simulink model "target_driver_2022_Ctrl_v_2_4_landing_2017a"  (R2024b)
settings: Solver=FixedStepDiscrete  StartTime=0.0  StopTime=13  FixedStep=0.0001  RelTol=1e-3  EnableMultiTasking=on
values from neighbouring files (symbols this model uses):
  A = gamma_2*gamma_3*Thrust_desired    [force2voltage.m]
  a2_lb = -0.25    [target_driver_setup_2022_Ctrl_V_2_4.m]    (also in target_driver_setup_2022_Ctrl_V_2_4_geometric.m; target_driver_setup_mpc_12msdelay.m; target_driver_setup_mpc_andWLQP.m)
  a2_openloop = -0    (= 0)    [target_driver_setup_2022_Ctrl_V_2_4.m]    (also in target_driver_setup_2022_Ctrl_V_2_4_geometric.m; target_driver_setup_mpc_12msdelay.m; target_driver_setup_mpc_andWLQP.m)
  a2_ub = 0.25    [target_driver_setup_2022_Ctrl_V_2_4.m]    (also in target_driver_setup_2022_Ctrl_V_2_4_geometric.m; target_driver_setup_mpc_12msdelay.m; target_driver_setup_mpc_andWLQP.m)
  adaptive_flag = 0    [target_driver_setup_2022_Ctrl_V_2_4.m]    (also in target_driver_setup_2022_Ctrl_V_2_4_geometric.m; target_driver_setup_mpc_12msdelay.m = 1; target_driver_setup_mpc_andWLQP.m = 1)
  adaptive_gain = [gamma_adaptive, adaptive_roll_limit, adaptive_pitch_limit, adaptive_yaw_limit, c_2_adaptive, gamma_lateral_adaptive, adaptive_x_limit, adaptive_y_limit, adaptive_z_limit, c_1_adaptive]    [target_driver_setup_2022_Ctrl_V_2_4.m]    (also in target_driver_setup_2022_Ctrl_V_2_4_geometric.m; target_driver_setup_mpc_12msdelay.m; target_driver_setup_mpc_andWLQP.m)
  adaptive_lateral_flag = 0    [target_driver_setup_2022_Ctrl_V_2_4.m]    (also in target_driver_setup_2022_Ctrl_V_2_4_geometric.m; target_driver_setup_mpc_12msdelay.m = 1; target_driver_setup_mpc_andWLQP.m = 1)
  adaptive_pitch_init = 0    [target_driver_setup_2022_Ctrl_V_2_4.m]    (also in target_driver_setup_2022_Ctrl_V_2_4_geometric.m; target_driver_setup_mpc_12msdelay.m; target_driver_setup_mpc_andWLQP.m)
  adaptive_pitch_limit = 0.1/(scale^2)    (= 1e-07)    [target_driver_setup_2022_Ctrl_V_2_4.m]    (also in target_driver_setup_2022_Ctrl_V_2_4_geometric.m = 3e-07; target_driver_setup_mpc_12msdelay.m; target_driver_setup_mpc_andWLQP.m)
  adaptive_pitch_limit_low = -adaptive_pitch_limit    (= -1e-07)    [target_driver_setup_2022_Ctrl_V_2_4.m]    (also in target_driver_setup_2022_Ctrl_V_2_4_geometric.m = -3e-07; target_driver_setup_mpc_12msdelay.m; target_driver_setup_mpc_andWLQP.m)
  adaptive_roll_init = 0    [target_driver_setup_2022_Ctrl_V_2_4.m]    (also in target_driver_setup_2022_Ctrl_V_2_4_geometric.m; target_driver_setup_mpc_12msdelay.m; target_driver_setup_mpc_andWLQP.m)
  adaptive_roll_limit = 0.3/(scale^2)    (= 3e-07)    [target_driver_setup_2022_Ctrl_V_2_4.m]    (also in target_driver_setup_2022_Ctrl_V_2_4_geometric.m; target_driver_setup_mpc_12msdelay.m; target_driver_setup_mpc_andWLQP.m)
  adaptive_roll_limit_low = -adaptive_roll_limit    (= -3e-07)    [target_driver_setup_2022_Ctrl_V_2_4.m]    (also in target_driver_setup_2022_Ctrl_V_2_4_geometric.m; target_driver_setup_mpc_12msdelay.m; target_driver_setup_mpc_andWLQP.m)
  adaptive_x_init = 0    [target_driver_setup_2022_Ctrl_V_2_4.m]    (also in target_driver_setup_2022_Ctrl_V_2_4_geometric.m; target_driver_setup_mpc_12msdelay.m; target_driver_setup_mpc_andWLQP.m)
  adaptive_x_limit = 0.15/(scale)    (= 0.00015)    [target_driver_setup_2022_Ctrl_V_2_4.m]    (also in target_driver_setup_2022_Ctrl_V_2_4_geometric.m = 7.5e-05; target_driver_setup_mpc_12msdelay.m; target_driver_setup_mpc_andWLQP.m)
  adaptive_x_limit_low = -adaptive_x_limit    (= -0.00015)    [target_driver_setup_2022_Ctrl_V_2_4.m]    (also in target_driver_setup_2022_Ctrl_V_2_4_geometric.m = -7.5e-05; target_driver_setup_mpc_12msdelay.m; target_driver_setup_mpc_andWLQP.m)
  adaptive_y_init = 0    [target_driver_setup_2022_Ctrl_V_2_4.m]    (also in target_driver_setup_2022_Ctrl_V_2_4_geometric.m; target_driver_setup_mpc_12msdelay.m; target_driver_setup_mpc_andWLQP.m)
  adaptive_y_limit = 0.15/(scale)    (= 0.00015)    [target_driver_setup_2022_Ctrl_V_2_4.m]    (also in target_driver_setup_2022_Ctrl_V_2_4_geometric.m = 7.5e-05; target_driver_setup_mpc_12msdelay.m; target_driver_setup_mpc_andWLQP.m)
  adaptive_y_limit_low = -adaptive_y_limit    (= -0.00015)    [target_driver_setup_2022_Ctrl_V_2_4.m]    (also in target_driver_setup_2022_Ctrl_V_2_4_geometric.m = -7.5e-05; target_driver_setup_mpc_12msdelay.m; target_driver_setup_mpc_andWLQP.m)
  adaptive_yaw_init = 0    [target_driver_setup_2022_Ctrl_V_2_4.m]    (also in target_driver_setup_2022_Ctrl_V_2_4_geometric.m; target_driver_setup_mpc_12msdelay.m; target_driver_setup_mpc_andWLQP.m)
  adaptive_yaw_limit = 0.035/(scale^2)    (= 3.5e-08)    [target_driver_setup_2022_Ctrl_V_2_4.m]    (also in target_driver_setup_2022_Ctrl_V_2_4_geometric.m; target_driver_setup_mpc_12msdelay.m; target_driver_setup_mpc_andWLQP.m)
  adaptive_yaw_limit_low = -adaptive_yaw_limit    (= -3.5e-08)    [target_driver_setup_2022_Ctrl_V_2_4.m]    (also in target_driver_setup_2022_Ctrl_V_2_4_geometric.m; target_driver_setup_mpc_12msdelay.m; target_driver_setup_mpc_andWLQP.m)
  adaptive_z_init = 0/scale    (= 0)    [target_driver_setup_2022_Ctrl_V_2_4.m]    (also in target_driver_setup_2022_Ctrl_V_2_4_geometric.m; target_driver_setup_mpc_12msdelay.m; target_driver_setup_mpc_andWLQP.m)
  adaptive_z_limit = 0.20/(scale)    (= 0.0002)    [target_driver_setup_2022_Ctrl_V_2_4.m]    (also in target_driver_setup_2022_Ctrl_V_2_4_geometric.m = 0.0008; target_driver_setup_mpc_12msdelay.m = 0.0008; target_driver_setup_mpc_andWLQP.m = 0.0008)
  adaptive_z_limit_low = -adaptive_z_limit/1    (= -0.0002)    [target_driver_setup_2022_Ctrl_V_2_4.m]    (also in target_driver_setup_2022_Ctrl_V_2_4_geometric.m = -0.0008; target_driver_setup_mpc_12msdelay.m = -0.0008; target_driver_setup_mpc_andWLQP.m = -0.0008)
  att_s = 500    [target_driver_setup_2022_Ctrl_V_2_4.m]    (also in target_driver_setup_2022_Ctrl_V_2_4_geometric.m; target_driver_setup_mpc_12msdelay.m; target_driver_setup_mpc_andWLQP.m)
  b_1_d_desired = [1,0,0]    [target_driver_setup_2022_Ctrl_V_2_4.m]    (also in target_driver_setup_2022_Ctrl_V_2_4_geometric.m; target_driver_setup_mpc_12msdelay.m; target_driver_setup_mpc_andWLQP.m)
  closedloop_flag = 1    [target_driver_setup_2022_Ctrl_V_2_4.m]    (also in target_driver_setup_2022_Ctrl_V_2_4_geometric.m = 0; target_driver_setup_mpc_12msdelay.m = 0; target_driver_setup_mpc_andWLQP.m = 0)
  control_gain = [k_x,k_v, k_R, k_Omega, k_z, k_vz, k_Rx]    [target_driver_setup_2022_Ctrl_V_2_4.m]    (also in target_driver_setup_2022_Ctrl_V_2_4_geometric.m = [k_x,k_v,k_R,k_Omega_pitch,k_Omega_roll,k_z,k_vz,k_Rx]; target_driver_setup_mpc_12msdelay.m = [k_x, k_v, k_R, k_Omega, k_z, k_vz, k_Rx,                  k; target_driver_setup_mpc_andWLQP.m = [k_x, k_v, k_R, k_Omega, k_z, k_vz, k_Rx,                  k)
  delay = delay-vicon_sample_cycle/2    [target_driver_setup_2022_Ctrl_V_2_4.m]    (also in target_driver_setup_2022_Ctrl_V_2_4_geometric.m; target_driver_setup_mpc_12msdelay.m; target_driver_setup_mpc_andWLQP.m)
  drv_amp = abs((vleft_p2p-vright_p2p))/2+min(vleft_p2p,vright_p2p)    [Wing_traj_to_Voltage.m]    (also in force2voltage.m; target_driver_setup_2022_Ctrl_V_2_4.m = 160; target_driver_setup_2022_Ctrl_V_2_4_geometric.m = 110; target_driver_setup_mpc_12msdelay.m = 150)
  drv_bias = max_drv_bias    (= 300)    [target_driver_setup_2022_Ctrl_V_2_4.m]    (also in target_driver_setup_2022_Ctrl_V_2_4_geometric.m = 200; target_driver_setup_mpc_12msdelay.m = 200; target_driver_setup_mpc_andWLQP.m = 200)
  drv_pitch_left = vleft_pitch    [Wing_traj_to_Voltage.m]    (also in force2voltage.m = 0; target_driver_setup_2022_Ctrl_V_2_4.m = 0; target_driver_setup_2022_Ctrl_V_2_4_geometric.m = 9.05; target_driver_setup_mpc_12msdelay.m = 9.05)
  drv_pitch_right = vright_pitch    [Wing_traj_to_Voltage.m]    (also in force2voltage.m = 0; target_driver_setup_2022_Ctrl_V_2_4.m = 0; target_driver_setup_2022_Ctrl_V_2_4_geometric.m = 9.05; target_driver_setup_mpc_12msdelay.m = 9.05)
  drv_roll = (vleft_p2p-vright_p2p)/4    [Wing_traj_to_Voltage.m]    (also in force2voltage.m; target_driver_setup_2022_Ctrl_V_2_4.m = -2; target_driver_setup_2022_Ctrl_V_2_4_geometric.m = -0.001; target_driver_setup_mpc_12msdelay.m = -0.001)
  f_fin = f    (= 155)    [target_driver_setup_2022_Ctrl_V_2_4.m]    (also in target_driver_setup_2022_Ctrl_V_2_4_geometric.m; target_driver_setup_mpc_12msdelay.m; target_driver_setup_mpc_andWLQP.m)
  f_int = f    (= 155)    [target_driver_setup_2022_Ctrl_V_2_4.m]    (also in target_driver_setup_2022_Ctrl_V_2_4_geometric.m; target_driver_setup_mpc_12msdelay.m; target_driver_setup_mpc_andWLQP.m)
  g = 9.8    [target_driver_setup_2022_Ctrl_V_2_4.m]    (also in target_driver_setup_2022_Ctrl_V_2_4_geometric.m; target_driver_setup_mpc_12msdelay.m; target_driver_setup_mpc_andWLQP.m = 9.81; test_full_attitude_mpc.m = 9.81)
  I_moment_vec = [Ixx, Iyy, Izz]    [target_driver_setup_2022_Ctrl_V_2_4.m]    (also in target_driver_setup_2022_Ctrl_V_2_4_geometric.m; target_driver_setup_mpc_12msdelay.m; target_driver_setup_mpc_andWLQP.m)
  landing_flag = 0    [target_driver_setup_2022_Ctrl_V_2_4.m]    (also in target_driver_setup_2022_Ctrl_V_2_4_geometric.m; target_driver_setup_mpc_12msdelay.m; target_driver_setup_mpc_andWLQP.m)
  landing_parameter = [start_delay+T,transition_rate, rising_time, falling_time, landing_rising_time, landing_z_decrease, landing_y_decrease, landing_x_decrease]    [target_driver_setup_2022_Ctrl_V_2_4.m]    (also in target_driver_setup_2022_Ctrl_V_2_4_geometric.m; target_driver_setup_mpc_12msdelay.m; target_driver_setup_mpc_andWLQP.m)
  low_bound = -8    [target_driver_setup_2022_Ctrl_V_2_4.m]    (also in target_driver_setup_2022_Ctrl_V_2_4_geometric.m = -5; target_driver_setup_mpc_12msdelay.m = -10; target_driver_setup_mpc_andWLQP.m = -10)
  low_bound_eR = -0.8    [target_driver_setup_2022_Ctrl_V_2_4.m]    (also in target_driver_setup_2022_Ctrl_V_2_4_geometric.m = -1.2; target_driver_setup_mpc_12msdelay.m = -1.2; target_driver_setup_mpc_andWLQP.m = -1.2)
  low_bound_vx = -0.5    [target_driver_setup_2022_Ctrl_V_2_4.m]    (also in target_driver_setup_2022_Ctrl_V_2_4_geometric.m; target_driver_setup_mpc_12msdelay.m; target_driver_setup_mpc_andWLQP.m)
  low_bound_vy = -0.5    [target_driver_setup_2022_Ctrl_V_2_4.m]    (also in target_driver_setup_2022_Ctrl_V_2_4_geometric.m; target_driver_setup_mpc_12msdelay.m; target_driver_setup_mpc_andWLQP.m)
  low_bound_vz = -0.5    [target_driver_setup_2022_Ctrl_V_2_4.m]    (also in target_driver_setup_2022_Ctrl_V_2_4_geometric.m; target_driver_setup_mpc_12msdelay.m; target_driver_setup_mpc_andWLQP.m)
  low_bound_x = -0.06    [target_driver_setup_2022_Ctrl_V_2_4.m]    (also in target_driver_setup_2022_Ctrl_V_2_4_geometric.m = -0.1; target_driver_setup_mpc_12msdelay.m = -0.6; target_driver_setup_mpc_andWLQP.m = -0.6)
  low_bound_y = -0.06    [target_driver_setup_2022_Ctrl_V_2_4.m]    (also in target_driver_setup_2022_Ctrl_V_2_4_geometric.m; target_driver_setup_mpc_12msdelay.m = -0.6; target_driver_setup_mpc_andWLQP.m = -0.6)
  low_bound_z = -0.04    [target_driver_setup_2022_Ctrl_V_2_4.m]    (also in target_driver_setup_2022_Ctrl_V_2_4_geometric.m; target_driver_setup_mpc_12msdelay.m = -0.1; target_driver_setup_mpc_andWLQP.m = -0.1)
  m = t <= t_zoom    [plot_roll_torque_cmd_vs_actual.m]    (also in plot_roll_torque_cmd_vs_actual_flightlog.m = t >= t0 & t <= t1; target_driver_setup_2022_Ctrl_V_2_4.m = 0.000124; target_driver_setup_2022_Ctrl_V_2_4_geometric.m = 8.5655e-05; target_driver_setup_mpc_12msdelay.m = 8.5655e-05)
  params_vec = [params_opt.delta_1, params_opt.delta_2, params_opt.delta_3,      params_opt.gamma_1, params_opt.gamma_2_1, params_opt.gamma_3,      params_opt.eta, params_opt.nu, params_opt.mu]'    [force2voltage_tuningSandbox.m]    (also in target_driver_setup_2022_Ctrl_V_2_4.m = [params_opt.delta_1, params_opt.delta_2, params_opt.delta_3,; target_driver_setup_2022_Ctrl_V_2_4_geometric.m = [params_opt.delta_1, params_opt.delta_2, params_opt.delta_3,; target_driver_setup_mpc_12msdelay.m = [params_opt.delta_1, params_opt.delta_2, params_opt.delta_3,; target_driver_setup_mpc_andWLQP.m = [params_opt.delta_1, params_opt.delta_2, params_opt.delta_3,)
  phase = 0    [target_driver_setup_2022_Ctrl_V_2_4.m]    (also in target_driver_setup_2022_Ctrl_V_2_4_geometric.m; target_driver_setup_mpc_12msdelay.m; target_driver_setup_mpc_andWLQP.m)
  r_desired = [default_x, default_y,z_desired]    [target_driver_setup_2022_Ctrl_V_2_4.m]    (also in target_driver_setup_2022_Ctrl_V_2_4_geometric.m; target_driver_setup_mpc_12msdelay.m; target_driver_setup_mpc_andWLQP.m)
  roll_offset_angle = 0    [target_driver_setup_2022_Ctrl_V_2_4.m]    (also in target_driver_setup_2022_Ctrl_V_2_4_geometric.m; target_driver_setup_mpc_12msdelay.m; target_driver_setup_mpc_andWLQP.m)
  running_time = start_delay+total_T    (= 8.5)    [target_driver_setup_2022_Ctrl_V_2_4.m]    (also in target_driver_setup_2022_Ctrl_V_2_4_geometric.m = 10; target_driver_setup_mpc_12msdelay.m = 0.5; target_driver_setup_mpc_andWLQP.m = 10)
  running_time_control = start_delay_control+total_T+0.0    (= 8.6)    [target_driver_setup_2022_Ctrl_V_2_4.m]    (also in target_driver_setup_2022_Ctrl_V_2_4_geometric.m = 10; target_driver_setup_mpc_12msdelay.m = 0.5; target_driver_setup_mpc_andWLQP.m = 10)
  start_delay = 2.0    (= 2)    [target_driver_setup_2022_Ctrl_V_2_4.m]    (also in target_driver_setup_2022_Ctrl_V_2_4_geometric.m = 0; target_driver_setup_mpc_12msdelay.m = 0; target_driver_setup_mpc_andWLQP.m = 0)
  start_delay_control = start_delay + ramp_delay    (= 2.1)    [target_driver_setup_2022_Ctrl_V_2_4.m]    (also in target_driver_setup_2022_Ctrl_V_2_4_geometric.m = 0; target_driver_setup_mpc_12msdelay.m = 0; target_driver_setup_mpc_andWLQP.m = 0)
  T = 0.5    [target_driver_setup_2022_Ctrl_V_2_4.m]    (also in target_driver_setup_2022_Ctrl_V_2_4_geometric.m = 10; target_driver_setup_mpc_12msdelay.m; target_driver_setup_mpc_andWLQP.m = 10; test_full_attitude_mpc.m = T0 + nu(1))
  task_flag = 0    [target_driver_setup_2022_Ctrl_V_2_4.m]    (also in target_driver_setup_2022_Ctrl_V_2_4_geometric.m; target_driver_setup_mpc_12msdelay.m; target_driver_setup_mpc_andWLQP.m)
  task_parameter = [radius_ref, frequency_ref, radius_ratio, lissajous_ratio, lissajous_delta, lissajous_amplitude_ratio,z_radius_ratio]    [target_driver_setup_2022_Ctrl_V_2_4.m]    (also in target_driver_setup_2022_Ctrl_V_2_4_geometric.m; target_driver_setup_mpc_12msdelay.m; target_driver_setup_mpc_andWLQP.m)
  upp_bound = 8    [target_driver_setup_2022_Ctrl_V_2_4.m]    (also in target_driver_setup_2022_Ctrl_V_2_4_geometric.m = 5; target_driver_setup_mpc_12msdelay.m = 10; target_driver_setup_mpc_andWLQP.m = 10)
  upp_bound_eR = 0.8    [target_driver_setup_2022_Ctrl_V_2_4.m]    (also in target_driver_setup_2022_Ctrl_V_2_4_geometric.m = 1.2; target_driver_setup_mpc_12msdelay.m = 1.2; target_driver_setup_mpc_andWLQP.m = 1.2)
  upp_bound_vx = 0.5    [target_driver_setup_2022_Ctrl_V_2_4.m]    (also in target_driver_setup_2022_Ctrl_V_2_4_geometric.m; target_driver_setup_mpc_12msdelay.m; target_driver_setup_mpc_andWLQP.m)
  upp_bound_vy = 0.5    [target_driver_setup_2022_Ctrl_V_2_4.m]    (also in target_driver_setup_2022_Ctrl_V_2_4_geometric.m; target_driver_setup_mpc_12msdelay.m; target_driver_setup_mpc_andWLQP.m)
  upp_bound_vz = 0.5    [target_driver_setup_2022_Ctrl_V_2_4.m]    (also in target_driver_setup_2022_Ctrl_V_2_4_geometric.m; target_driver_setup_mpc_12msdelay.m; target_driver_setup_mpc_andWLQP.m)
  upp_bound_x = 0.06    [target_driver_setup_2022_Ctrl_V_2_4.m]    (also in target_driver_setup_2022_Ctrl_V_2_4_geometric.m = 0.1; target_driver_setup_mpc_12msdelay.m = 0.6; target_driver_setup_mpc_andWLQP.m = 0.6)
  upp_bound_y = 0.06    [target_driver_setup_2022_Ctrl_V_2_4.m]    (also in target_driver_setup_2022_Ctrl_V_2_4_geometric.m; target_driver_setup_mpc_12msdelay.m = 0.6; target_driver_setup_mpc_andWLQP.m = 0.6)
  upp_bound_z = 0.04    [target_driver_setup_2022_Ctrl_V_2_4.m]    (also in target_driver_setup_2022_Ctrl_V_2_4_geometric.m; target_driver_setup_mpc_12msdelay.m = 0.1; target_driver_setup_mpc_andWLQP.m = 0.1)
undefined symbols (not defined in the file or in its folder): Com1, DiscIntNeverNeededParam, left_mapping, left_mapping_F_to_Phi, lp_den, lp_num, none, right_mapping, right_mapping_F_to_Phi, vlp_den, vlp_num
libraries: simulink x32, xpcseriallib x6, xpcnilib x3, xpcutilitieslib x3
(part 4 of 7)

== system target_driver_2022_Ctrl_v_2_4_landing_2017a/Desired attitude and normalized error/saturated normalized error observation/saturated normalized altitude error  ==
  averaged velocity : Inport
  averaged position : Inport  Port=2
  "r_desired " : Inport  Port=3
  v_desired : Inport  Port=4
  Demux{,1..3} (4 alike) : Demux  Outputs=3
  Gain1 : Gain  Gain=2/(upp_bound_y-low_bound_y)
  Gain2 : Gain  Gain=2/(upp_bound_x-low_bound_x)
  Gain3 : Gain  Gain=2/(upp_bound_vx-low_bound_vx)
  Gain4 : Gain  Gain=2/(upp_bound_vy-low_bound_vy)
  Gain5 : Gain  Gain=2/(upp_bound_z-low_bound_z)
  Gain9 : Gain  Gain=2/(upp_bound_vz-low_bound_vz)
  Mux : Mux  Inputs=3
  Mux1 : Mux  Inputs=3
  Saturation1 : Saturate  UpperLimit=upp_bound_y  LowerLimit=low_bound_y
  Saturation2 : Saturate  UpperLimit=upp_bound_x  LowerLimit=low_bound_x
  Saturation3 : Saturate  UpperLimit=upp_bound_z  LowerLimit=low_bound_z
  Saturation4 : Saturate  UpperLimit=upp_bound_vx  LowerLimit=low_bound_vx
  Saturation5 : Saturate  UpperLimit=upp_bound_vz  LowerLimit=low_bound_vz
  Saturation6 : Saturate  UpperLimit=upp_bound_vy  LowerLimit=low_bound_vy
  Sum{,1..5} (6 alike) : Sum  Inputs=+-
  Position error : Outport
  velocity_error : Outport  Port=2
  wires:
  Demux2/3 -> Sum/2
  Sum/1 -> Saturation3/1
  Sum1/1 -> Saturation5/1
  Gain5/1 -> Mux/3
  Saturation3/1 -> Gain5/1
  Saturation5/1 -> Gain9/1
  Gain9/1 -> Mux1/3
  Mux1/1 -> velocity_error/1
  averaged velocity/1 -> Demux1/1
  averaged position/1 -> Demux/1
  Demux/3 -> Sum/1
  Demux1/3 -> Sum1/1
  "r_desired "/1 -> Demux2/1
  Saturation1/1 -> Gain1/1
  Sum2/1 -> Saturation1/1
  Demux2/2 -> Sum2/2
  Demux/2 -> Sum2/1
  Sum3/1 -> Saturation2/1
  Saturation2/1 -> Gain2/1
  Demux/1 -> Sum3/1
  Demux2/1 -> Sum3/2
  v_desired/1 -> Demux3/1
  Demux3/3 -> Sum1/2
  Saturation4/1 -> Gain3/1
  Gain3/1 -> Mux1/1
  Sum4/1 -> Saturation4/1
  Demux3/1 -> Sum4/2
  Demux1/1 -> Sum4/1
  Saturation6/1 -> Gain4/1
  Gain4/1 -> Mux1/2
  Sum5/1 -> Saturation6/1
  Demux3/2 -> Sum5/2
  Demux1/2 -> Sum5/1
  Gain2/1 -> Mux/1
  Gain1/1 -> Mux/2
  Mux/1 -> Position error/1

== system target_driver_2022_Ctrl_v_2_4_landing_2017a/Observer for averaged system/Attitude Observer/Geometric Averaging Rotation Matix ==
  note: Geometric mean in SO(3)
      | 1) Output the Geometric average over one cycle (n=4 samples: 500Hz vicon sampling and 160Hz flapping signal)
      |
      | Patrick 2021 Mar
  Vicon Update flag : Inport
  Current Rotation : Inport  Port=2
  Averaged quaternion : MATLAB Function  TreatAsAtomicUnit=on
  Delay6 : Delay  DelayLength=1  InitialCondition=0
  Demux3 : Demux
  Demux4 : Demux
  Geometric Averaging Rotation M : Subsystem
  Mux3 : Mux
  Mux4 : Mux
  Raw quaternion : MATLAB Function  TreatAsAtomicUnit=on
  Averaged quaternion output : Outport
  "Averaged Rotation Matrix " : Outport  Port=2
  "Raw quaternion output " : Outport  Port=3
  Previous Averaged Rotation Matrix : Outport  Port=4
  wires:
  Raw quaternion/1(quat) -> Demux4/1
  Demux4/3 -> Mux4/3
  Demux4/4 -> Mux4/4
  Demux4/1 -> Mux4/1
  Demux4/2 -> Mux4/2
  Mux4/1 -> "Raw quaternion output "/1
  Vicon Update flag/1 -> Geometric Averaging Rotation M/2(Vicon Update)
  Current Rotation/1 -> Raw quaternion/1(R), Geometric Averaging Rotation M/1("Current Rotation ")
  Mux3/1 -> Averaged quaternion output/1
  Demux3/4 -> Mux3/4
  Averaged quaternion/1(quat) -> Demux3/1
  Demux3/3 -> Mux3/3
  Geometric Averaging Rotation M/1(Averaged Rotation Matrix) -> Delay6/1, Averaged quaternion/1(R), "Averaged Rotation Matrix "/1
  Demux3/2 -> Mux3/2
  Demux3/1 -> Mux3/1
  Delay6/1 -> Geometric Averaging Rotation M/3("Previous Averaged Rotation "), Previous Averaged Rotation Matrix/1

== system target_driver_2022_Ctrl_v_2_4_landing_2017a/Observer for averaged system/Attitude Observer/Geometric derivative in SO(3) ==
  note: First order geometric derivative in SO(3)
      | Patrick 2021 Mar
  Previous Averaged Rotation M : Inport
  Vicon Count : Inport  Port=2
  Current Averaged Rotation M : Inport  Port=3
  "Vicon Update Flag " : Inport  Port=4
  Demux2 : Demux  Outputs=3
  "First order geometric derivative in SO(3) " : MATLAB Function  TreatAsAtomicUnit=on
  Mux2 : Mux  Inputs=3
  Previous Omega : Delay  DelayLength=1  InitialCondition=0
  filtered derivative5 : Subsystem
  Filtered Geometric derivative in SO(3) : Outport
  wires:
  Previous Omega/1 -> "First order geometric derivative in SO(3) "/3(omega_prev)
  Previous Averaged Rotation M/1 -> "First order geometric derivative in SO(3) "/1(R_prev)
  Demux2/1 -> Mux2/1
  Demux2/2 -> Mux2/2
  filtered derivative5/1(Out1) -> Demux2/1
  Mux2/1 -> Filtered Geometric derivative in SO(3)/1
  "First order geometric derivative in SO(3) "/1(omega) -> Previous Omega/1, filtered derivative5/1(In1)
  Demux2/3 -> Mux2/3
  "Vicon Update Flag "/1 -> "First order geometric derivative in SO(3) "/4(update)
  Current Averaged Rotation M/1 -> "First order geometric derivative in SO(3) "/2(R_cur)
  Vicon Count/1 -> "First order geometric derivative in SO(3) "/5(count)

== system target_driver_2022_Ctrl_v_2_4_landing_2017a/Observer for averaged system/Euler derivative & filtered angular velocity /filtered derivative ==
  In1 : Inport
  att_s : Gain  Gain=att_s
  filtered derivative : simulink/Discrete/Transfer Fcn Lead or Lag  PoleZ=k_da  ZeroZ=1  ICPrevOutput=0.0  ICPrevInput=0.0  DoSatur=off
  low pass3 : DiscreteTransferFcn  Numerator=lp_num  Denominator=lp_den
  Out1 : Outport
  wires:
  att_s/1 -> filtered derivative/1
  In1/1 -> att_s/1
  low pass3/1 -> Out1/1
  filtered derivative/1 -> low pass3/1

== system target_driver_2022_Ctrl_v_2_4_landing_2017a/Observer for averaged system/Position Observer/LowPassFiltere1 ==
  In1 : Inport
  low pass3 : DiscreteTransferFcn  Numerator=lp_num  Denominator=lp_den
  Out1 : Outport
  wires:
  low pass3/1 -> Out1/1
  In1/1 -> low pass3/1

== system target_driver_2022_Ctrl_v_2_4_landing_2017a/Observer for averaged system/Position Observer/LowPassFiltere2 ==
  In1 : Inport
  low pass3 : DiscreteTransferFcn  Numerator=lp_num  Denominator=lp_den
  Out1 : Outport
  wires:
  low pass3/1 -> Out1/1
  In1/1 -> low pass3/1

== system target_driver_2022_Ctrl_v_2_4_landing_2017a/Observer for averaged system1/Attitude Observer/Geometric Averaging Rotation Matix ==
  note: Geometric mean in SO(3)
      | 1) Output the Geometric average over one cycle (n=4 samples: 500Hz vicon sampling and 160Hz flapping signal)
      |
      | Patrick 2021 Mar
  Vicon Update flag : Inport
  Current Rotation : Inport  Port=2
  Averaged quaternion : MATLAB Function  TreatAsAtomicUnit=on
  Delay6 : Delay  DelayLength=1  InitialCondition=0
  Demux3 : Demux
  Demux4 : Demux
  Geometric Averaging Rotation M : Subsystem
  Mux3 : Mux
  Mux4 : Mux
  Raw quaternion : MATLAB Function  TreatAsAtomicUnit=on
  Averaged quaternion output : Outport
  "Averaged Rotation Matrix " : Outport  Port=2
  "Raw quaternion output " : Outport  Port=3
  Previous Averaged Rotation Matrix : Outport  Port=4
  wires:
  Raw quaternion/1(quat) -> Demux4/1
  Demux4/3 -> Mux4/3
  Demux4/4 -> Mux4/4
  Demux4/1 -> Mux4/1
  Demux4/2 -> Mux4/2
  Mux4/1 -> "Raw quaternion output "/1
  Vicon Update flag/1 -> Geometric Averaging Rotation M/2(Vicon Update)
  Current Rotation/1 -> Raw quaternion/1(R), Geometric Averaging Rotation M/1("Current Rotation ")
  Mux3/1 -> Averaged quaternion output/1
  Demux3/4 -> Mux3/4
  Averaged quaternion/1(quat) -> Demux3/1
  Demux3/3 -> Mux3/3
  Geometric Averaging Rotation M/1(Averaged Rotation Matrix) -> Delay6/1, Averaged quaternion/1(R), "Averaged Rotation Matrix "/1
  Demux3/2 -> Mux3/2
  Demux3/1 -> Mux3/1
  Delay6/1 -> Geometric Averaging Rotation M/3("Previous Averaged Rotation "), Previous Averaged Rotation Matrix/1

== system target_driver_2022_Ctrl_v_2_4_landing_2017a/Observer for averaged system1/Attitude Observer/Geometric derivative in SO(3) ==
  note: First order geometric derivative in SO(3)
      | Patrick 2021 Mar
  Previous Averaged Rotation M : Inport
  Vicon Count : Inport  Port=2
  Current Averaged Rotation M : Inport  Port=3
  "Vicon Update Flag " : Inport  Port=4
  Demux2 : Demux  Outputs=3
  "First order geometric derivative in SO(3) " : MATLAB Function  TreatAsAtomicUnit=on
  Mux2 : Mux  Inputs=3
  Previous Omega : Delay  DelayLength=1  InitialCondition=0
  filtered derivative5 : Subsystem
  Filtered Geometric derivative in SO(3) : Outport
  wires:
  Previous Omega/1 -> "First order geometric derivative in SO(3) "/3(omega_prev)
  Previous Averaged Rotation M/1 -> "First order geometric derivative in SO(3) "/1(R_prev)
  Demux2/1 -> Mux2/1
  Demux2/2 -> Mux2/2
  filtered derivative5/1(Out1) -> Demux2/1
  Mux2/1 -> Filtered Geometric derivative in SO(3)/1
  "First order geometric derivative in SO(3) "/1(omega) -> Previous Omega/1, filtered derivative5/1(In1)
  Demux2/3 -> Mux2/3
  "Vicon Update Flag "/1 -> "First order geometric derivative in SO(3) "/4(update)
  Current Averaged Rotation M/1 -> "First order geometric derivative in SO(3) "/2(R_cur)
  Vicon Count/1 -> "First order geometric derivative in SO(3) "/5(count)

== system target_driver_2022_Ctrl_v_2_4_landing_2017a/Observer for averaged system1/Euler derivative & filtered angular velocity /filtered derivative ==
  In1 : Inport
  att_s : Gain  Gain=att_s
  filtered derivative : simulink/Discrete/Transfer Fcn Lead or Lag  PoleZ=k_da  ZeroZ=1  ICPrevOutput=0.0  ICPrevInput=0.0  DoSatur=off
  low pass3 : DiscreteTransferFcn  Numerator=lp_num  Denominator=lp_den
  Out1 : Outport
  wires:
  att_s/1 -> filtered derivative/1
  In1/1 -> att_s/1
  low pass3/1 -> Out1/1
  filtered derivative/1 -> low pass3/1

== system target_driver_2022_Ctrl_v_2_4_landing_2017a/Observer for averaged system1/Position Observer/LowPassFiltere1 ==
  In1 : Inport
  low pass3 : DiscreteTransferFcn  Numerator=lp_num  Denominator=lp_den
  Out1 : Outport
  wires:
  low pass3/1 -> Out1/1
  In1/1 -> low pass3/1

== system target_driver_2022_Ctrl_v_2_4_landing_2017a/Observer for averaged system1/Position Observer/LowPassFiltere2 ==
  In1 : Inport
  low pass3 : DiscreteTransferFcn  Numerator=lp_num  Denominator=lp_den
  Out1 : Outport
  wires:
  low pass3/1 -> Out1/1
  In1/1 -> low pass3/1

== system target_driver_2022_Ctrl_v_2_4_landing_2017a/Plant/signal generator a3/Bias_Signal ==
  note: time constant = 0.002sec
  QuasiEnable : Inport
  BiasVolts : Inport  Port=2
  AveragedBias : Subsystem
  PreGain : Gain
  Product : Product  RndMeth=Zero
  SIgnalForRamp_binary : Subsystem
  SaturatingRamp : DiscreteIntegrator  gainval=10  SampleTime=-1  LimitOutput=on  UpperSaturationLimit=1  LowerSaturationLimit=0  ICPrevOutput=DiscIntNeverNeededParam  ICPrevScaledInput=DiscIntNeverNeededParam
  BiasD2A : Outport
  wires:
  PreGain/1 -> BiasD2A/1
  BiasVolts/1 -> AveragedBias/1(In1)
  QuasiEnable/1 -> SIgnalForRamp_binary/1(In1)
  SIgnalForRamp_binary/1(Out1) -> SaturatingRamp/1
  SaturatingRamp/1 -> Product/1
  AveragedBias/1(Out1) -> Product/2
  Product/1 -> PreGain/1

== system target_driver_2022_Ctrl_v_2_4_landing_2017a/Plant/signal generator a3/Drive_Signal ==
  QuasiEnable : Inport
  Frequency : Inport  Port=2
  Offset : Inport  Port=3
  Amplitude : Inport  Port=4
  PitchBias : Inport  Port=5
  Phase : Inport  Port=6
  "a2 " : Inport  Port=7
  AveragedAmp_filtered : Subsystem
  AveragedOffset_filtered : Subsystem
  FlattenedSine1 : Subsystem
  FlattenedSine_phase : Subsystem  Commented=on
  OutputWithRamping : Product  RndMeth=Zero
  PreGain : Constant
  PrescaledAmp : Product  RndMeth=Zero
  PrescaledOffset : Product  RndMeth=Zero
  ProductPhase : Product  RndMeth=Zero
  ProductPhase1 : Product  RndMeth=Zero
  RampUpOrDown : DiscreteIntegrator  gainval=10  SampleTime=-1  LimitOutput=on  UpperSaturationLimit=1  LowerSaturationLimit=0  ICPrevOutput=DiscIntNeverNeededParam  ICPrevScaledInput=DiscIntNeverNeededParam
  SignalForRamp_binary : Subsystem
  SignalForSin_binary : Subsystem
  Sinewave : Subsystem  Commented=on
  Sum : Sum
  Sum1 : Sum
  signal with gain : Product  RndMeth=Zero
  SignalOutput : Outport
  WithoutRamp : Outport  Port=2
  RampOutput : Outport  Port=3
  AmplitudeOutput : Outport  Port=4
  OffsetOutput : Outport  Port=5
  WithoutRamp1 : Outport  Port=6
  wires:
  OutputWithRamping/1 -> SignalOutput/1
  Sum/1 -> WithoutRamp/1, OutputWithRamping/2
  PrescaledOffset/1 -> AveragedOffset_filtered/1(In1)
  AveragedAmp_filtered/1(Out1) -> AmplitudeOutput/1, signal with gain/2
  PrescaledAmp/1 -> AveragedAmp_filtered/1(In1)
  "a2 "/1 -> FlattenedSine1/3(a2)
  ProductPhase/1 -> FlattenedSine1/1(freq)
  ProductPhase1/1 -> WithoutRamp1/1
  Offset/1 -> Sum1/1
  AveragedOffset_filtered/1(Out1) -> OffsetOutput/1, Sum/2
  signal with gain/1 -> Sum/1
  SignalForSin_binary/1(Out1) -> ProductPhase1/1, ProductPhase/1
  Amplitude/1 -> PrescaledAmp/1
  Sum1/1 -> PrescaledOffset/1
  Frequency/1 -> ProductPhase/2
  PreGain/1 -> PrescaledAmp/2, PrescaledOffset/2
  FlattenedSine1/1(split cycle signal) -> signal with gain/1
  QuasiEnable/1 -> SignalForRamp_binary/1(In1)
  SignalForRamp_binary/1(Out1) -> RampUpOrDown/1
  Phase/1 -> ProductPhase1/2, FlattenedSine1/2(phase)
  PitchBias/1 -> Sum1/2
  RampUpOrDown/1 -> SignalForSin_binary/1(In1), RampOutput/1, OutputWithRamping/1

== system target_driver_2022_Ctrl_v_2_4_landing_2017a/Plant/signal generator a3/Drive_Signal1 ==
  QuasiEnable : Inport
  Frequency : Inport  Port=2
  Offset : Inport  Port=3
  Amplitude : Inport  Port=4
  PitchBias : Inport  Port=5
  a2 : Inport  Port=6
  AveragedAmp_filtered : Subsystem
  AveragedOffset_filtered : Subsystem
  FlattenedSine1 : Subsystem
  OutputWithRamping : Product  RndMeth=Zero
  PreGain : Constant
  PrescaledAmp : Product  RndMeth=Zero
  PrescaledOffset : Product  RndMeth=Zero
  ProductPhase : Product  RndMeth=Zero
  RampUpOrDown : DiscreteIntegrator  gainval=10  SampleTime=-1  LimitOutput=on  UpperSaturationLimit=1  LowerSaturationLimit=0  ICPrevOutput=DiscIntNeverNeededParam  ICPrevScaledInput=DiscIntNeverNeededParam
  SignalForRamp_binary : Subsystem
  SignalForSin_binary : Subsystem
  Sine Wave : Subsystem  Commented=on
  Sum : Sum
  Sum1 : Sum
  signal with gain : Product  RndMeth=Zero
  SignalOutput : Outport
  WithoutRamp : Outport  Port=2
  RampOutput : Outport  Port=3
  AmplitudeOutput : Outport  Port=4
  OffsetOutput : Outport  Port=5
  wires:
  PrescaledAmp/1 -> AveragedAmp_filtered/1(In1)
  Sum/1 -> OutputWithRamping/2, WithoutRamp/1
  RampUpOrDown/1 -> RampOutput/1, OutputWithRamping/1, SignalForSin_binary/1(In1)
  QuasiEnable/1 -> SignalForRamp_binary/1(In1)
  SignalForRamp_binary/1(Out1) -> RampUpOrDown/1
  signal with gain/1 -> Sum/1
  Frequency/1 -> ProductPhase/2
  SignalForSin_binary/1(Out1) -> ProductPhase/1
  AveragedOffset_filtered/1(Out1) -> Sum/2, OffsetOutput/1
  PrescaledOffset/1 -> AveragedOffset_filtered/1(In1)
  PreGain/1 -> PrescaledAmp/2, PrescaledOffset/2
  OutputWithRamping/1 -> SignalOutput/1
  AveragedAmp_filtered/1(Out1) -> signal with gain/2, AmplitudeOutput/1
  Sum1/1 -> PrescaledOffset/1
  Offset/1 -> Sum1/1
  PitchBias/1 -> Sum1/2
  Amplitude/1 -> PrescaledAmp/1
  ProductPhase/1 -> FlattenedSine1/1(freq)
  FlattenedSine1/1(split cycle signal) -> signal with gain/1
  a2/1 -> FlattenedSine1/2(a2)

== system target_driver_2022_Ctrl_v_2_4_landing_2017a/Plant/signal generator a3/SignalSaturationLimit ==
  BiasMax : Inport
  SignalRaw : Inport  Port=2
  GainBias : Gain
  MaxOf : MinMax  Function=max  Inputs=2
  MinOf : MinMax  Inputs=2
  ground : Constant
  SignalSatd : Outport
  wires:
  BiasMax/1 -> GainBias/1
  SignalRaw/1 -> MinOf/2
  MinOf/1 -> MaxOf/1
  MaxOf/1 -> SignalSatd/1
  GainBias/1 -> MinOf/1
  ground/1 -> MaxOf/2

== system target_driver_2022_Ctrl_v_2_4_landing_2017a/Plant/signal generator a3/SignalSaturationLimit1 ==
  BiasMax : Inport
  SignalRaw : Inport  Port=2
  GainBias : Gain
  MaxOf : MinMax  Function=max  Inputs=2
  MinOf : MinMax  Inputs=2
  ground : Constant
  SignalSatd : Outport
  wires:
  BiasMax/1 -> GainBias/1
  SignalRaw/1 -> MinOf/2
  MinOf/1 -> MaxOf/1
  MaxOf/1 -> SignalSatd/1
  GainBias/1 -> MinOf/1
  ground/1 -> MaxOf/2

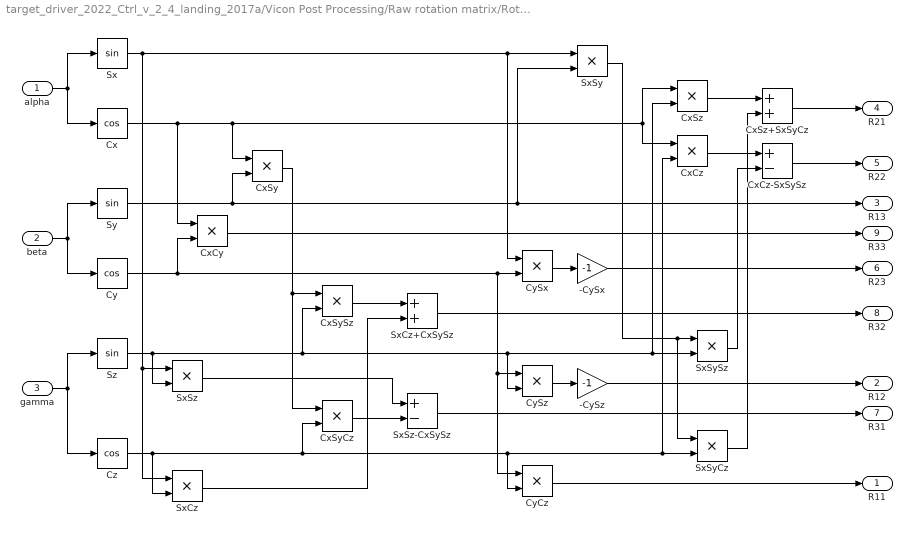
== system target_driver_2022_Ctrl_v_2_4_landing_2017a/Vicon Post Processing/Raw rotation matrix/Rotation Matrix ==
  alpha : Inport
  beta : Inport  Port=2
  gamma : Inport  Port=3
  -CySx : Gain  Gain=-1
  -CySz : Gain  Gain=-1
  Cx : Trigonometry  Operator=cos
  CxCy : Product  RndMeth=Zero
  CxCz : Product  RndMeth=Zero
  CxCz-SxSySz : Sum  Inputs=+-
  CxSy : Product  RndMeth=Zero
  CxSyCz : Product  RndMeth=Zero
  CxSySz : Product  RndMeth=Zero
  CxSz : Product  RndMeth=Zero
  CxSz+SxSyCz : Sum
  Cy : Trigonometry  Operator=cos
  CyCz : Product  RndMeth=Zero
  CySx : Product  RndMeth=Zero
  CySz : Product  RndMeth=Zero
  Cz : Trigonometry  Operator=cos
  Sx : Trigonometry
  SxCz : Product  RndMeth=Zero
  SxCz+CxSySz : Sum
  SxSy : Product  RndMeth=Zero
  SxSyCz : Product  RndMeth=Zero
  SxSySz : Product  RndMeth=Zero
  SxSz : Product  RndMeth=Zero
  SxSz-CxSySz : Sum  Inputs=+-
  Sy : Trigonometry
  Sz : Trigonometry
  R11 : Outport
  R12 : Outport  Port=2
  R13 : Outport  Port=3
  R21 : Outport  Port=4
  R22 : Outport  Port=5
  R23 : Outport  Port=6
  R31 : Outport  Port=7
  R32 : Outport  Port=8
  R33 : Outport  Port=9
  wires:
  beta/1 -> Sy/1, Cy/1
  alpha/1 -> Sx/1, Cx/1
  Sy/1 -> R13/1, SxSy/2, CxSy/2
  Cy/1 -> CySx/2, CySz/1, CyCz/1, CxCy/2
  CySx/1 -> -CySx/1
  -CySx/1 -> R23/1
  gamma/1 -> Sz/1, Cz/1
  Sx/1 -> CySx/1, SxSy/1, SxCz/1, SxSz/1
  SxSy/1 -> SxSyCz/1, SxSySz/1
  Sz/1 -> SxSySz/2, CxSz/2, CySz/2, CxSySz/2, SxSz/2
  Cz/1 -> SxSyCz/2, CxCz/2, CyCz/2, CxSyCz/2, SxCz/2
  Cx/1 -> CxSz/1, CxCz/1, CxSy/1, CxCy/1
  SxSyCz/1 -> CxSz+SxSyCz/2
  CxSz/1 -> CxSz+SxSyCz/1
  CxCz/1 -> CxCz-SxSySz/1
  SxSySz/1 -> CxCz-SxSySz/2
  CySz/1 -> -CySz/1
  CyCz/1 -> R11/1
  -CySz/1 -> R12/1
  CxSz+SxSyCz/1 -> R21/1
  CxCz-SxSySz/1 -> R22/1
  CxSy/1 -> CxSySz/1, CxSyCz/1
  CxSySz/1 -> SxCz+CxSySz/1
  SxCz/1 -> SxCz+CxSySz/2
  CxSyCz/1 -> SxSz-CxSySz/2
  SxSz/1 -> SxSz-CxSySz/1
  SxSz-CxSySz/1 -> R31/1
  SxCz+CxSySz/1 -> R32/1
  CxCy/1 -> R33/1

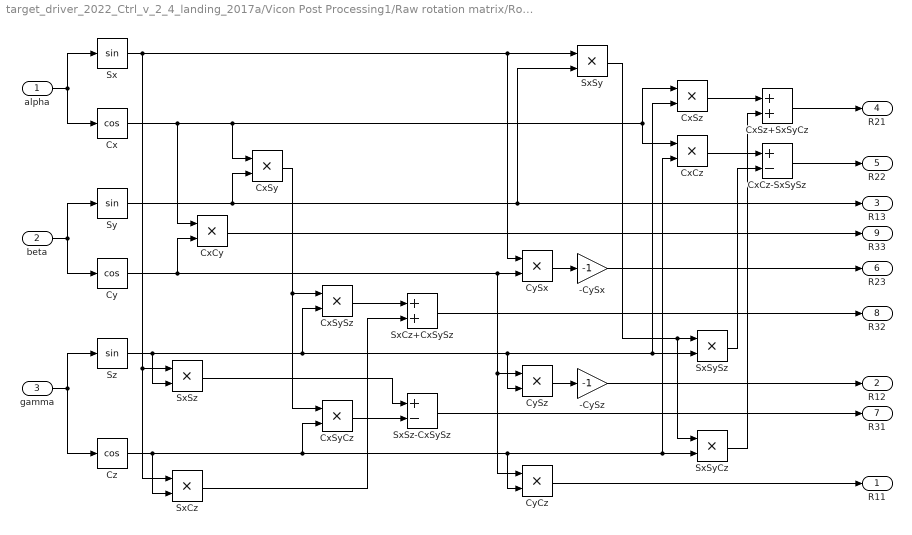
== system target_driver_2022_Ctrl_v_2_4_landing_2017a/Vicon Post Processing1/Raw rotation matrix/Rotation Matrix ==
  alpha : Inport
  beta : Inport  Port=2
  gamma : Inport  Port=3
  -CySx : Gain  Gain=-1
  -CySz : Gain  Gain=-1
  Cx : Trigonometry  Operator=cos
  CxCy : Product  RndMeth=Zero
  CxCz : Product  RndMeth=Zero
  CxCz-SxSySz : Sum  Inputs=+-
  CxSy : Product  RndMeth=Zero
  CxSyCz : Product  RndMeth=Zero
  CxSySz : Product  RndMeth=Zero
  CxSz : Product  RndMeth=Zero
  CxSz+SxSyCz : Sum
  Cy : Trigonometry  Operator=cos
  CyCz : Product  RndMeth=Zero
  CySx : Product  RndMeth=Zero
  CySz : Product  RndMeth=Zero
  Cz : Trigonometry  Operator=cos
  Sx : Trigonometry
  SxCz : Product  RndMeth=Zero
  SxCz+CxSySz : Sum
  SxSy : Product  RndMeth=Zero
  SxSyCz : Product  RndMeth=Zero
  SxSySz : Product  RndMeth=Zero
  SxSz : Product  RndMeth=Zero
  SxSz-CxSySz : Sum  Inputs=+-
  Sy : Trigonometry
  Sz : Trigonometry
  R11 : Outport
  R12 : Outport  Port=2
  R13 : Outport  Port=3
  R21 : Outport  Port=4
  R22 : Outport  Port=5
  R23 : Outport  Port=6
  R31 : Outport  Port=7
  R32 : Outport  Port=8
  R33 : Outport  Port=9
  wires:
  beta/1 -> Sy/1, Cy/1
  alpha/1 -> Sx/1, Cx/1
  Sy/1 -> R13/1, SxSy/2, CxSy/2
  Cy/1 -> CySx/2, CySz/1, CyCz/1, CxCy/2
  CySx/1 -> -CySx/1
  -CySx/1 -> R23/1
  gamma/1 -> Sz/1, Cz/1
  Sx/1 -> CySx/1, SxSy/1, SxCz/1, SxSz/1
  SxSy/1 -> SxSyCz/1, SxSySz/1
  Sz/1 -> SxSySz/2, CxSz/2, CySz/2, CxSySz/2, SxSz/2
  Cz/1 -> SxSyCz/2, CxCz/2, CyCz/2, CxSyCz/2, SxCz/2
  Cx/1 -> CxSz/1, CxCz/1, CxSy/1, CxCy/1
  SxSyCz/1 -> CxSz+SxSyCz/2
  CxSz/1 -> CxSz+SxSyCz/1
  CxCz/1 -> CxCz-SxSySz/1
  SxSySz/1 -> CxCz-SxSySz/2
  CySz/1 -> -CySz/1
  CyCz/1 -> R11/1
  -CySz/1 -> R12/1
  CxSz+SxSyCz/1 -> R21/1
  CxCz-SxSySz/1 -> R22/1
  CxSy/1 -> CxSySz/1, CxSyCz/1
  CxSySz/1 -> SxCz+CxSySz/1
  SxCz/1 -> SxCz+CxSySz/2
  CxSyCz/1 -> SxSz-CxSySz/2
  SxSz/1 -> SxSz-CxSySz/1
  SxSz-CxSySz/1 -> R31/1
  SxCz+CxSySz/1 -> R32/1
  CxCy/1 -> R33/1

== system target_driver_2022_Ctrl_v_2_4_landing_2017a/closed loop signal generator/Bias_Signal/AveragedBias ==
  note: To avoid having signal "jump",
      | we want SMOOTH transitions
      | in frequency (i.e., a weighted sum
      | of current freq and freq some delta t ago)
  note: time constant = 0.002sec
  In1 : Inport
  Discrete Transfer Fcn : DiscreteTransferFcn  Numerator=[0.05]  Denominator=[1 -.95]
  Out1 : Outport
  wires:
  In1/1 -> Discrete Transfer Fcn/1
  Discrete Transfer Fcn/1 -> Out1/1

== system target_driver_2022_Ctrl_v_2_4_landing_2017a/closed loop signal generator/Bias_Signal/SIgnalForRamp_binary ==
  note: Should output 1 or -1,
      | so signal ramps UP to 1
      | or DOWN to 0.
  In1 : Inport
  Add : Sum  Inputs=+-
  Compare To Zero : simulink/Logic and Bit Operations/Compare To Zero  relop=>  OutDataTypeStr=uint8  ZeroCross=off
  Constant : Constant
  Data Type Conversion : DataTypeConversion  OutDataTypeStr=double  SaturateOnIntegerOverflow=off  RndMeth=Floor
  Gain : Gain  Gain=2
  Out1 : Outport
  wires:
  In1/1 -> Compare To Zero/1
  Compare To Zero/1 -> Data Type Conversion/1
  Gain/1 -> Add/1
  Constant/1 -> Add/2
  Add/1 -> Out1/1
  Data Type Conversion/1 -> Gain/1

== system target_driver_2022_Ctrl_v_2_4_landing_2017a/closed loop signal generator/Left Drive Signal /AveragedAmp_filtered ==
  note: To avoid having signal "jump",
      | we want SMOOTH transitions
      | in frequency (i.e., a weighted sum
      | of current freq and freq some delta t ago)
  note: time constant 0.002sec
      | for 10kHz samping
  In1 : Inport
  Discrete Transfer Fcn : DiscreteTransferFcn  Numerator=[0.05]  Denominator=[1 -.95]
  Out1 : Outport
  wires:
  In1/1 -> Discrete Transfer Fcn/1
  Discrete Transfer Fcn/1 -> Out1/1

== system target_driver_2022_Ctrl_v_2_4_landing_2017a/closed loop signal generator/Left Drive Signal /AveragedOffset_filtered ==
  note: To avoid having signal "jump",
      | we want SMOOTH transitions
      | in frequency (i.e., a weighted sum
      | of current freq and freq some delta t ago)
  note: c
  note: time constant 0.02sec
      | for 10kHz samping
  In1 : Inport
  Discrete Transfer Fcn : DiscreteTransferFcn  Numerator=[0.05]  Denominator=[1 -.95]
  Out1 : Outport
  wires:
  In1/1 -> Discrete Transfer Fcn/1
  Discrete Transfer Fcn/1 -> Out1/1

== system target_driver_2022_Ctrl_v_2_4_landing_2017a/closed loop signal generator/Left Drive Signal /FlattenedSine ==
  In2 : Inport
  In1 : Inport  Port=2
  0.1 : Gain  Gain=0.1
  1.1 : Gain  Gain=1.1
  2pi : Gain  Gain=2*pi
  3f : Gain  Gain=3
  Add : Sum
  Add1 : Sum
  first harmonic : Trigonometry  OutputSignalType=real
  integrate(omega*t) : DiscreteIntegrator  SampleTime=-1  ICPrevOutput=DiscIntNeverNeededParam  ICPrevScaledInput=DiscIntNeverNeededParam
  third harmonic : Trigonometry  OutputSignalType=real
  split cycle signal : Outport
  wires:
  In2/1 -> 2pi/1
  2pi/1 -> integrate(omega*t)/1
  integrate(omega*t)/1 -> Add1/2
  3f/1 -> third harmonic/1
  first harmonic/1 -> 1.1/1
  third harmonic/1 -> 0.1/1
  1.1/1 -> Add/1
  0.1/1 -> Add/2
  Add/1 -> split cycle signal/1
  In1/1 -> Add1/1
  Add1/1 -> 3f/1, first harmonic/1

== system target_driver_2022_Ctrl_v_2_4_landing_2017a/closed loop signal generator/Left Drive Signal /FlattenedSine_phase ==
  f : Inport
  phase : Inport  Port=2
  0.1 : Gain  Gain=0.1
  1.1 : Gain  Gain=1.1
  2pi : Gain  Gain=2*pi
  3f : Gain  Gain=3
  Add : Sum
  Sum : Sum  Inputs=|++
  first harmonic : Trigonometry  OutputSignalType=real
  integrate(omega*t) : DiscreteIntegrator  SampleTime=-1  ICPrevOutput=DiscIntNeverNeededParam  ICPrevScaledInput=DiscIntNeverNeededParam
  pi/180 : Gain  Gain=pi/180
  third harmonic : Trigonometry  OutputSignalType=real
  split cycle signal : Outport
  wires:
  f/1 -> 2pi/1
  2pi/1 -> integrate(omega*t)/1
  3f/1 -> third harmonic/1
  first harmonic/1 -> 1.1/1
  third harmonic/1 -> 0.1/1
  1.1/1 -> Add/1
  0.1/1 -> Add/2
  Add/1 -> split cycle signal/1
  Sum/1 -> first harmonic/1, 3f/1
  pi/180/1 -> Sum/2
  integrate(omega*t)/1 -> Sum/1
  phase/1 -> pi/180/1

== system target_driver_2022_Ctrl_v_2_4_landing_2017a/closed loop signal generator/Left Drive Signal /SignalForRamp_binary ==
  note: Should output 1 or -1,
      | so signal ramps UP to 1
      | or DOWN to 0.
  In1 : Inport
  Add : Sum  Inputs=+-
  Compare To Zero : simulink/Logic and Bit Operations/Compare To Zero  relop=>  OutDataTypeStr=uint8  ZeroCross=off
  Constant : Constant
  Data Type Conversion : DataTypeConversion  OutDataTypeStr=double  SaturateOnIntegerOverflow=off  RndMeth=Floor
  Gain : Gain  Gain=2
  Out1 : Outport
  wires:
  In1/1 -> Compare To Zero/1
  Compare To Zero/1 -> Data Type Conversion/1
  Gain/1 -> Add/1
  Constant/1 -> Add/2
  Add/1 -> Out1/1
  Data Type Conversion/1 -> Gain/1

== system target_driver_2022_Ctrl_v_2_4_landing_2017a/closed loop signal generator/Left Drive Signal /SignalForSin_binary ==
  note: We want this to stay "high" for 1
      | second after the actual "enable"
      | is turned off...
  In1 : Inport
  Compare To Zero : simulink/Logic and Bit Operations/Compare To Zero  relop=>  OutDataTypeStr=uint8  ZeroCross=off
  Data Type Conversion : DataTypeConversion  OutDataTypeStr=double  SaturateOnIntegerOverflow=off  RndMeth=Floor
  Out1 : Outport
  wires:
  In1/1 -> Compare To Zero/1
  Compare To Zero/1 -> Data Type Conversion/1
  Data Type Conversion/1 -> Out1/1

== system target_driver_2022_Ctrl_v_2_4_landing_2017a/closed loop signal generator/Left Drive Signal /Sinewave ==
  In2 : Inport
  2pi : Gain  Gain=2*pi
  first harmonic : Trigonometry  OutputSignalType=real
  integrate(omega*t) : DiscreteIntegrator  SampleTime=-1  ICPrevOutput=DiscIntNeverNeededParam  ICPrevScaledInput=DiscIntNeverNeededParam
  split cycle signal : Outport
  wires:
  In2/1 -> 2pi/1
  2pi/1 -> integrate(omega*t)/1
  integrate(omega*t)/1 -> first harmonic/1
  first harmonic/1 -> split cycle signal/1

== system target_driver_2022_Ctrl_v_2_4_landing_2017a/closed loop signal generator/Right Drive Signal/AveragedAmp_filtered ==
  note: To avoid having signal "jump",
      | we want SMOOTH transitions
      | in frequency (i.e., a weighted sum
      | of current freq and freq some delta t ago)
  note: time constant 0.002sec
      | for 10kHz samping
  In1 : Inport
  Discrete Transfer Fcn : DiscreteTransferFcn  Numerator=[0.05]  Denominator=[1 -.95]
  Out1 : Outport
  wires:
  In1/1 -> Discrete Transfer Fcn/1
  Discrete Transfer Fcn/1 -> Out1/1

== system target_driver_2022_Ctrl_v_2_4_landing_2017a/closed loop signal generator/Right Drive Signal/AveragedOffset_filtered ==
  note: To avoid having signal "jump",
      | we want SMOOTH transitions
      | in frequency (i.e., a weighted sum
      | of current freq and freq some delta t ago)
  note: c
  note: time constant 0.02sec
      | for 10kHz samping
  In1 : Inport
  Discrete Transfer Fcn : DiscreteTransferFcn  Numerator=[0.05]  Denominator=[1 -.95]
  Out1 : Outport
  wires:
  In1/1 -> Discrete Transfer Fcn/1
  Discrete Transfer Fcn/1 -> Out1/1

== system target_driver_2022_Ctrl_v_2_4_landing_2017a/closed loop signal generator/Right Drive Signal/FlattenedSine ==
  In2 : Inport
  0.1 : Gain  Gain=0.1
  1.1 : Gain  Gain=1.1
  2pi : Gain  Gain=2*pi
  3f : Gain  Gain=3
  Add : Sum
  first harmonic : Trigonometry  OutputSignalType=real
  integrate(omega*t) : DiscreteIntegrator  SampleTime=-1  ICPrevOutput=DiscIntNeverNeededParam  ICPrevScaledInput=DiscIntNeverNeededParam
  third harmonic : Trigonometry  OutputSignalType=real
  split cycle signal : Outport
  wires:
  In2/1 -> 2pi/1
  2pi/1 -> integrate(omega*t)/1
  integrate(omega*t)/1 -> first harmonic/1, 3f/1
  3f/1 -> third harmonic/1
  first harmonic/1 -> 1.1/1
  third harmonic/1 -> 0.1/1
  1.1/1 -> Add/1
  0.1/1 -> Add/2
  Add/1 -> split cycle signal/1

== system target_driver_2022_Ctrl_v_2_4_landing_2017a/closed loop signal generator/Right Drive Signal/SignalForRamp_binary ==
  note: Should output 1 or -1,
      | so signal ramps UP to 1
      | or DOWN to 0.
  In1 : Inport
  Add : Sum  Inputs=+-
  Compare To Zero : simulink/Logic and Bit Operations/Compare To Zero  relop=>  OutDataTypeStr=uint8  ZeroCross=off
  Constant : Constant
  Data Type Conversion : DataTypeConversion  OutDataTypeStr=double  SaturateOnIntegerOverflow=off  RndMeth=Floor
  Gain : Gain  Gain=2
  Out1 : Outport
  wires:
  In1/1 -> Compare To Zero/1
  Compare To Zero/1 -> Data Type Conversion/1
  Gain/1 -> Add/1
  Constant/1 -> Add/2
  Add/1 -> Out1/1
  Data Type Conversion/1 -> Gain/1

== system target_driver_2022_Ctrl_v_2_4_landing_2017a/closed loop signal generator/Right Drive Signal/SignalForSin_binary ==
  note: We want this to stay "high" for 1
      | second after the actual "enable"
      | is turned off...
  In1 : Inport
  Compare To Zero : simulink/Logic and Bit Operations/Compare To Zero  relop=>  OutDataTypeStr=uint8  ZeroCross=off
  Data Type Conversion : DataTypeConversion  OutDataTypeStr=double  SaturateOnIntegerOverflow=off  RndMeth=Floor
  Out1 : Outport
  wires:
  In1/1 -> Compare To Zero/1
  Compare To Zero/1 -> Data Type Conversion/1
  Data Type Conversion/1 -> Out1/1

== system target_driver_2022_Ctrl_v_2_4_landing_2017a/closed loop signal generator/Right Drive Signal/Sine Wave ==
  In2 : Inport
  2pi : Gain  Gain=2*pi
  first harmonic : Trigonometry  OutputSignalType=real
  integrate(omega*t) : DiscreteIntegrator  SampleTime=-1  ICPrevOutput=DiscIntNeverNeededParam  ICPrevScaledInput=DiscIntNeverNeededParam
  split cycle signal : Outport
  wires:
  In2/1 -> 2pi/1
  2pi/1 -> integrate(omega*t)/1
  integrate(omega*t)/1 -> first harmonic/1
  first harmonic/1 -> split cycle signal/1

== system target_driver_2022_Ctrl_v_2_4_landing_2017a/signal generator a1/Bias_Signal/AveragedBias ==
  note: To avoid having signal "jump",
      | we want SMOOTH transitions
      | in frequency (i.e., a weighted sum
      | of current freq and freq some delta t ago)
  note: time constant = 0.002sec
  In1 : Inport
  Discrete Transfer Fcn : DiscreteTransferFcn  Numerator=[0.05]  Denominator=[1 -.95]
  Out1 : Outport
  wires:
  In1/1 -> Discrete Transfer Fcn/1
  Discrete Transfer Fcn/1 -> Out1/1

== system target_driver_2022_Ctrl_v_2_4_landing_2017a/signal generator a1/Bias_Signal/SIgnalForRamp_binary ==
  note: Should output 1 or -1,
      | so signal ramps UP to 1
      | or DOWN to 0.
  In1 : Inport
  Add : Sum  Inputs=+-
  Compare To Zero : simulink/Logic and Bit Operations/Compare To Zero  relop=>  OutDataTypeStr=uint8  ZeroCross=off
  Constant : Constant
  Data Type Conversion : DataTypeConversion  OutDataTypeStr=double  SaturateOnIntegerOverflow=off  RndMeth=Floor
  Gain : Gain  Gain=2
  Out1 : Outport
  wires:
  In1/1 -> Compare To Zero/1
  Compare To Zero/1 -> Data Type Conversion/1
  Gain/1 -> Add/1
  Constant/1 -> Add/2
  Add/1 -> Out1/1
  Data Type Conversion/1 -> Gain/1

== system target_driver_2022_Ctrl_v_2_4_landing_2017a/signal generator a1/Drive_Signal/AveragedAmp_filtered ==
  note: To avoid having signal "jump",
      | we want SMOOTH transitions
      | in frequency (i.e., a weighted sum
      | of current freq and freq some delta t ago)
  note: time constant 0.002sec
      | for 10kHz samping
  In1 : Inport
  Discrete Transfer Fcn : DiscreteTransferFcn  Numerator=[0.05]  Denominator=[1 -.95]
  Out1 : Outport
  wires:
  In1/1 -> Discrete Transfer Fcn/1
  Discrete Transfer Fcn/1 -> Out1/1

== system target_driver_2022_Ctrl_v_2_4_landing_2017a/signal generator a1/Drive_Signal/AveragedOffset_filtered ==
  note: To avoid having signal "jump",
      | we want SMOOTH transitions
      | in frequency (i.e., a weighted sum
      | of current freq and freq some delta t ago)
  note: c
  note: time constant 0.02sec
      | for 10kHz samping
  In1 : Inport
  Discrete Transfer Fcn : DiscreteTransferFcn  Numerator=[0.05]  Denominator=[1 -.95]
  Out1 : Outport
  wires:
  In1/1 -> Discrete Transfer Fcn/1
  Discrete Transfer Fcn/1 -> Out1/1

== system target_driver_2022_Ctrl_v_2_4_landing_2017a/signal generator a1/Drive_Signal/FlattenedSine1 ==
  freq : Inport
  phase : Inport  Port=2
  a2 : Inport  Port=3
  0.1 : Gain  Gain=0.1
  1.1 : Gain  Gain=1.1
  2f : Gain  Gain=2
  2pi : Gain  Gain=2*pi
  3f : Gain  Gain=3
  Add : Sum  Inputs=+++
  Add1 : Sum
  Amplitude Correction : Subsystem  Commented=on
  AveragedAmp_filtered : Subsystem
  Product : Product
  first harmonic : Trigonometry  OutputSignalType=real
  integrate(omega*t) : DiscreteIntegrator  SampleTime=-1  ICPrevOutput=DiscIntNeverNeededParam  ICPrevScaledInput=DiscIntNeverNeededParam
  second harmonic : Trigonometry  OutputSignalType=real
  third harmonic : Trigonometry  OutputSignalType=real
  split cycle signal : Outport
  wires:
  freq/1 -> 2pi/1
  2pi/1 -> integrate(omega*t)/1
  3f/1 -> third harmonic/1
  first harmonic/1 -> 1.1/1
  third harmonic/1 -> 0.1/1
  1.1/1 -> Add/1
  Add1/1 -> first harmonic/1, 2f/1, 3f/1
  integrate(omega*t)/1 -> Add1/1
  phase/1 -> Add1/2
  2f/1 -> second harmonic/1
  0.1/1 -> Add/2
  Product/1 -> Add/3
  second harmonic/1 -> Product/1
  Add/1 -> split cycle signal/1
  a2/1 -> AveragedAmp_filtered/1(In1)
  AveragedAmp_filtered/1(Out1) -> Product/2
